simulink subsystem "Autonomous_sub"  (R2023b)
settings: Solver=VariableStepAuto  StartTime=0.0  StopTime=10.0  RelTol=1e-3
undefined symbols (not defined in the file): Spline_Num_Poses_default, Spline_Ref_Poses_default
settings Model: Creator=ander  LastModifiedBy=ander

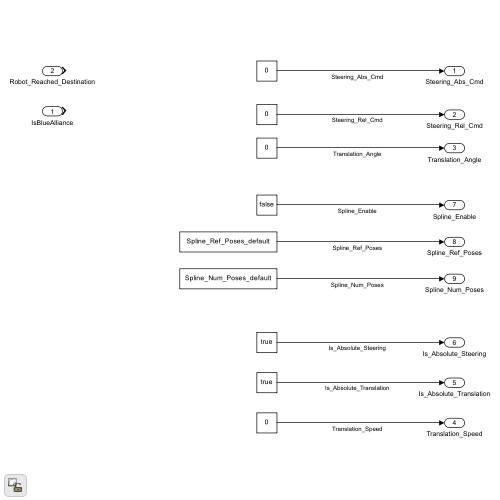
[thumbnail: Simulink's stored preview of the top-level diagram]
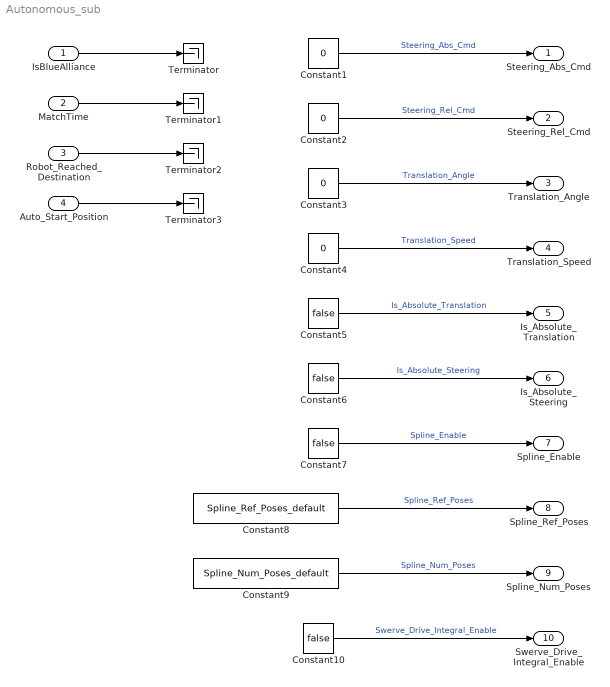
== system Autonomous_sub ==
  IsBlueAlliance : Inport
  MatchTime : Inport  Port=2
  Robot_Reached_Destination : Inport  Port=3
  Auto_Start_Position : Inport  Port=4
  Constant{1..4} (4 alike) : Constant  Value=0
  Constant10 : Constant  Value=false  OutDataTypeStr=boolean
  Constant5 : Constant  Value=false
  Constant6 : Constant  Value=false
  Constant7 : Constant  Value=false  OutDataTypeStr=boolean
  Constant8 : Constant  Value=Spline_Ref_Poses_default
  Constant9 : Constant  Value=Spline_Num_Poses_default  OutDataTypeStr=double
  Terminator{,1..3} (4 alike) : Terminator
  Steering_Abs_Cmd : Outport
  Steering_Rel_Cmd : Outport  Port=2
  Translation_Angle : Outport  Port=3
  Translation_Speed : Outport  Port=4
  Is_Absolute_Translation : Outport  Port=5
  Is_Absolute_Steering : Outport  Port=6
  Spline_Enable : Outport  Port=7
  Spline_Ref_Poses : Outport  Port=8
  Spline_Num_Poses : Outport  Port=9
  Swerve_Drive_Integral_Enable : Outport  Port=10
  wires:
  Constant9/1 -> Spline_Num_Poses/1  "Spline_Num_Poses"
  Constant10/1 -> Swerve_Drive_Integral_Enable/1  "Swerve_Drive_Integral_Enable"
  Constant8/1 -> Spline_Ref_Poses/1  "Spline_Ref_Poses"
  Constant1/1 -> Steering_Abs_Cmd/1  "Steering_Abs_Cmd"
  Constant2/1 -> Steering_Rel_Cmd/1  "Steering_Rel_Cmd"
  Constant4/1 -> Translation_Speed/1  "Translation_Speed"
  Constant3/1 -> Translation_Angle/1  "Translation_Angle"
  Constant6/1 -> Is_Absolute_Steering/1  "Is_Absolute_Steering"
  Constant7/1 -> Spline_Enable/1  "Spline_Enable"
  Constant5/1 -> Is_Absolute_Translation/1  "Is_Absolute_Translation"
  IsBlueAlliance/1 -> Terminator/1
  MatchTime/1 -> Terminator1/1
  Robot_Reached_Destination/1 -> Terminator2/1
  Auto_Start_Position/1 -> Terminator3/1
